simulink model "conv_test"  (R2024b)
settings: Solver=VariableStepAuto  StartTime=0.0  StopTime=5  RelTol=1e-3
values from neighbouring files (symbols this model uses):
  BinaryMessage = reshape(BinaryMessage,1,[])    [MessageInput.m]
  Frame_number = 32767    [MessageInput.m]
libraries: commdigbbndpm3 x2, commcnvcod2 x2, simulink x2, commchan3 x1
settings Model: Creator=fredr  LastModifiedBy=fredr

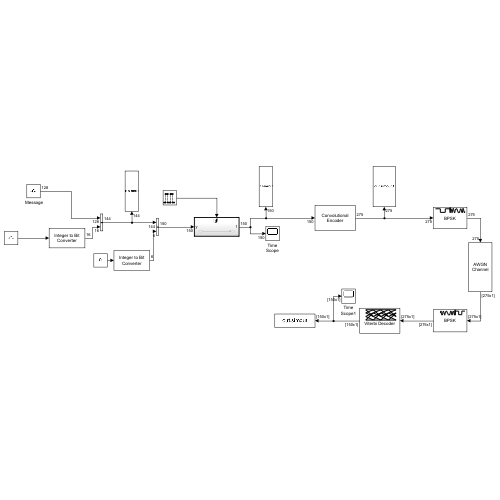
[thumbnail: Simulink's stored preview of the top-level diagram]
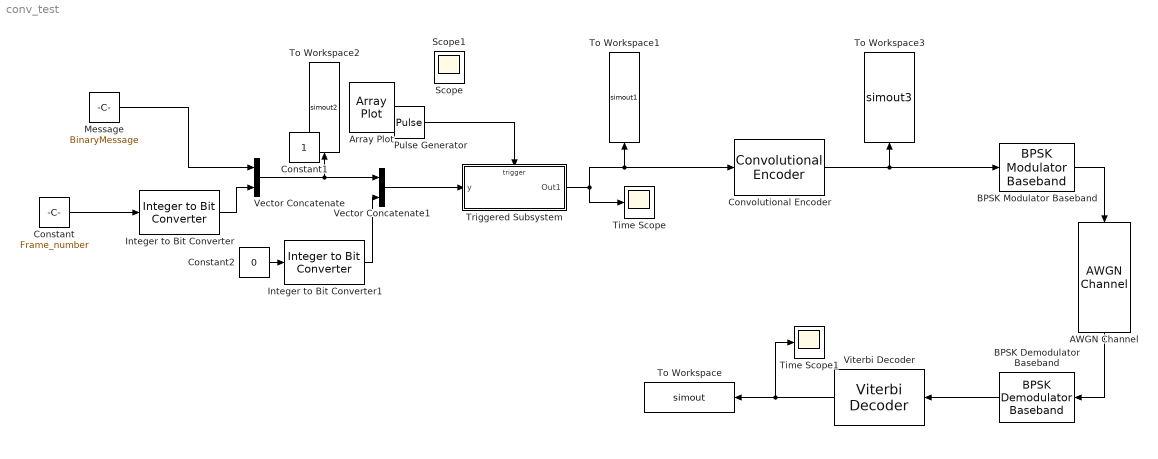
== system conv_test ==
  " Message" : Constant  Value=BinaryMessage
  AWGN Channel : commchan3/AWGN Channel  LegacyMode=off  NoiseMethod="Signal to noise ratio  (SNR)"  noiseMode="Signal to noise ratio  (SNR)"  EbNo=10  EsNo=10  SNR=10  BitsPerSymbol=1  SignalPower=1  SamplesPerSymbol=1  SymbolPeriod=1  VarianceSource=Parameter  Variance=1  RandomStream=Global stream  Seed=67  SimulateUsing=Code generation
  BPSK Demodulator Baseband : commdigbbndpm3/BPSK Demodulator Baseband  DecType=Hard decision  VarSource=Dialog  Variance=1  Ph=0  outDtype=Inherit via internal rule  derotateFactorWordLen=16  derotateFactorDataTypeStr=Inherit: Same word length as input  derotateFactorLastDataTypeStr=Inherit: Same word length as input
      settings: LibrarySourceBlock=|
      | commhdldigbbndpm/BPSK
      | Demodulator
      | Baseband
  BPSK Modulator Baseband : commdigbbndpm3/BPSK Modulator Baseband  Ph=0  outDtype=double  outWordLen=16  outUDDataType=sfix(16)  outFracLenMode=Best precision  outFracLen=15  outDataTypeStr=double  outLastDataTypeStr=double
      settings: LibrarySourceBlock=|
      | commhdldigbbndpm/BPSK
      | Modulator
      | Baseband
  Constant : Constant  Value=Frame_number
  Constant2 : Constant  Value=0
  Convolutional Encoder : commcnvcod2/Convolutional Encoder  trellis=poly2trellis(5, [23 35])  opMode=Continuous  DelayedResetAction=on  hasIniStPort=off  hasFinStPort=off  usePuncVector=on  punctureVector=P2  reset=Unused parameter value
      settings: LibrarySourceBlock=|
      | commhdlcnvcod/Convolutional
      | Encoder
  Integer to Bit Converter : simulink/Logic and Bit Operations/Integer to Bit Converter  nbits=16  signedInputValues=Unsigned  bitOrder=MSB first  outDtype=Inherit via internal rule
  Integer to Bit Converter1 : simulink/Logic and Bit Operations/Integer to Bit Converter  nbits=6  signedInputValues=Unsigned  bitOrder=MSB first  outDtype=Inherit via internal rule
  Pulse Generator : DiscretePulseGenerator
  Time Scope : Scope
  Time Scope1 : Scope
  To Workspace : ToWorkspace  VariableName=simout  SampleTime=-1
      settings: Save2DSignal=2-D array (concatenate along first dimension)
  To Workspace1 : ToWorkspace  VariableName=simout1  SampleTime=-1
      settings: Save2DSignal=2-D array (concatenate along first dimension)
  To Workspace2 : ToWorkspace  VariableName=simout2  SampleTime=-1
      settings: Save2DSignal=2-D array (concatenate along first dimension)
  To Workspace3 : ToWorkspace  VariableName=simout3  SampleTime=-1
      settings: Save2DSignal=2-D array (concatenate along first dimension)
  Triggered Subsystem : Subsystem  TreatAsAtomicUnit=on
  Vector Concatenate : Concatenate
  Vector Concatenate1 : Concatenate
  Viterbi Decoder : commcnvcod2/Viterbi Decoder  trellis=poly2trellis(5, [23 35])  isPunctured=on  punctureVector=P2  erasures=off  dectype=Hard decision  nsdecb=2  runSigValErrCheck=off  tbdepth=20  opmode=Continuous  reset=off  delayedResetAction=on  smWordLength=16  outDataType=double
      settings: LibrarySourceBlock=commhdlcnvcod/Viterbi Decoder
  Array Plot : ArrayPlot  IOType=viewer  IsFloating=on  WindowPosition=[609.000000,57.000000,800.000000,500.000000,]  ScopeFrameLocation=window  YLimits=[-10 10]  DefaultConfigurationName=dsp.scopes.ArrayPlotBlockSpecification
  Constant1 : Constant  IOType=siggen
  Scope : Scope
  Scope1 : Scope
  wires:
  Viterbi Decoder/1 -> Time Scope1/1, To Workspace/1
  BPSK Demodulator Baseband/1 -> Viterbi Decoder/1
  AWGN Channel/1 -> BPSK Demodulator Baseband/1
  BPSK Modulator Baseband/1 -> AWGN Channel/1
  Pulse Generator/1 -> Triggered Subsystem/Trigger
  Constant/1 -> Integer to Bit Converter/1
  " Message"/1 -> Vector Concatenate/1
  Integer to Bit Converter/1 -> Vector Concatenate/2
  Triggered Subsystem/1(Out1) -> Convolutional Encoder/1, To Workspace1/1, Time Scope/1
  Integer to Bit Converter1/1 -> Vector Concatenate1/2
  Vector Concatenate/1 -> To Workspace2/1, Vector Concatenate1/1
  Vector Concatenate1/1 -> Triggered Subsystem/1(y)
  Constant2/1 -> Integer to Bit Converter1/1
  Convolutional Encoder/1 -> BPSK Modulator Baseband/1, To Workspace3/1

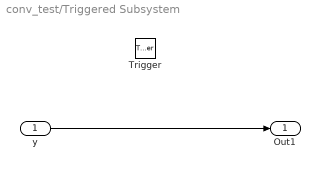
== system conv_test/Triggered Subsystem ==
  y : Inport
  Trigger : TriggerPort  VariantControl=(inherit)
  Out1 : Outport
  wires:
  y/1 -> Out1/1
